simulink model "simulink_part"  (R2016a)
settings: Solver=VariableStepAuto  StartTime=0.0  StopTime=1  RelTol=1e-3
libraries: powerlib x6, powerlib_meascontrol x6
settings Model: Creator=ziad abdelhamed  LastModifiedBy=ziad abdelhamed

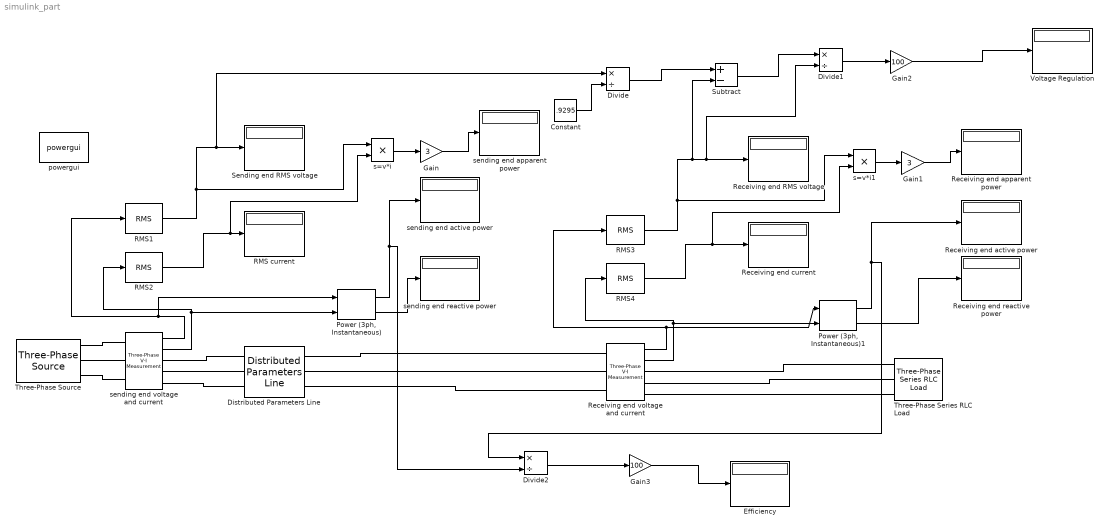
== system simulink_part ==
  Constant : Constant  Value=.9295
  Distributed Parameters Line : powerlib/Elements/Distributed Parameters Line  Phases=3  Frequency=60  Resistance=[.05 .05]  Inductance=[0.97e-3 .99e-3]  Capacitance=[11.5e-9 11.5e-9]  Length=300  x1=[8.73114913702011e-11 617530 617530;376.991118430775 376.991118430775 376.991118430775;1.18918707880175 0.426861843081656 -1.14393448371324]  x2=[1.60089247853505e-10 485242.976182768 485242.976182767;376.991118430775 376.991118430775 376.991118430775;-0.612639506584876 0.174011595737851 -1.39678473105705]  x3=[1.48338818762908e-12 1106.67820606831 1106.67820606832;376.991118430775 376.991118430775 376.991118430775;-2.38866595647793 1.209216979252 -0.361579347542891]  x4=[1.45080507751676e-12 3320.58863195203 3320.58863195202;376.991118430775 376.991118430775 376.991118430775;0.308585693257765 -0.174792776282672 -1.74558910307757]  x5=0.00101224996912818  V1=[8.731e-11 6.175e+05 6.175e+05;377 377 377;1.189 0.4269 -1.144]  V2=[1.601e-10 4.852e+05 4.852e+05;377 377 377;-0.6126 0.174 -1.397]  I1=[1.483e-12 1107 1107;377 377 377;-2.389 1.209 -0.3616]  I2=[1.451e-12 3321 3321;377 377 377;0.3086 -0.1748 -1.746]  nHarmo=1  Measurements=None
  Divide : Product  Inputs=*/
  Divide1 : Product  Inputs=*/
  Divide2 : Product  Inputs=*/
  "Efficiency " : Display
  Gain : Gain  Gain=3
  Gain1 : Gain  Gain=3
  Gain2 : Gain  Gain=100
  Gain3 : Gain  Gain=100
  "Power (3ph, Instantaneous)" : powerlib_meascontrol/Measurements/Power (3ph, Instantaneous)
  "Power (3ph, Instantaneous)1" : powerlib_meascontrol/Measurements/Power (3ph, Instantaneous)
  "RMS current " : Display
  RMS{1..4} (4 alike) : powerlib_meascontrol/Measurements/RMS  TrueRMS=on  Freq=60  RMSInit=0  Ts=0
  Receiving end RMS voltage : Display
  Receiving end active power : Display
  "Receiving end apparent power " : Display
  Receiving end current : Display
  "Receiving end reactive power " : Display
  Receiving end voltage and current : powerlib/Measurements/Three-Phase V-I Measurement  VoltageMeasurement=phase-to-ground  SetLabelV=off  LabelV=Vabc  Vpu=off  VpuLL=off  CurrentMeasurement=yes  SetLabelI=off  LabelI=Iabc  Ipu=off  Pbase=100e6  Vbase=500e3  OutputType=Complex  PhasorSimulation=off  PSBequivalent=0
  Sending end RMS voltage : Display
  Subtract : Sum  Inputs=+-
  Three-Phase Series RLC Load : powerlib/Elements/Three-Phase Series RLC Load  LConnTagsString=A|B|C  Configuration=Y (grounded)  NominalVoltage=500e3  Vabc=[1e3 1e3 1e3]  Vabcp=[1e3 1e3 1e3]  NominalFrequency=60  UnbalancedPower=off  ActivePower=800e6  InductivePower=600e6  CapacitivePower=0  Pabc=[10e3 9e3 11e3]  QLabc=[100 90 110]  QCabc=[100 90 110]  Pabcp=[10e3 9e3 11e3]  QLabcp=[100 90 110]  QCabcp=[100 90 110]  Measurements=None  LoadType=constant Z
  Three-Phase Source : powerlib/Electrical Sources/Three-Phase Source  InternalConnection=Yg  VoltagePhases=off  Voltage=617.53e3  PhaseAngle=16.1  Voltage_phases=[25e3 25e3 25e3]/sqrt(3)  PhaseAngles_phases=[0 -120 +120]  Frequency=60  NonIdealSource=off  SpecifyImpedance=off  Resistance=0.8929  Inductance=16.58e-3  ShortCircuitLevel=100e6  BaseVoltage=25e3  XRratio=7  BusType=swing  Pref=10e3  Qref=0  Prefabc=[10e3, 10e3, 10e3]  Qrefabc=[0, 0, 0]  Qmin=-inf  Qmax=inf
  "Voltage Regulation " : Display
  powergui : powerlib/powergui  Priority=1  SimulationMode=Continuous  SolverType=Tustin/Backward Euler (TBE)  SampleTime=50e-6  frequency=60  SPID=off  DisableSnubberDevices=off  DisableRonSwitches=off  DisableVfSwitches=off  SwTol=0  DisplayEquations=off  Interpol=off  ExternalGateDelay=off  methode=off  Ts=10  FunctionMessages=off  echomessages=off  HookPort=off  EnableUseOfTLC=off  x0status=blocks  frequencyindice=60  Pbase=100e6  ErrMax=1e-4  Iterations=50  UnitsV=kV  UnitsW=MW  buscounter=0  RestoreLinks=warning  ResistiveCurrentMeasurement=off  Frange=[0:2:500]  Ylog=off  Xlog=on  ShowGrid=off  save=off  variable=ZData  structure=0  ZoomFFT=off  StartTime=0.0  cycles=1  DisplayStyle=1  fundamental=60  FreqAxis=off  MaxFrequency=1000  frequencyindicesteady=1  RmsSteady=1  display=off
  s=v*i : Product
  s=v*i1 : Product
  sending end active power : Display
  "sending end apparent power " : Display
  sending end reactive power : Display
  "sending end voltage and current " : powerlib/Measurements/Three-Phase V-I Measurement  VoltageMeasurement=phase-to-ground  SetLabelV=off  LabelV=Vabc  Vpu=off  VpuLL=off  CurrentMeasurement=yes  SetLabelI=off  LabelI=Iabc  Ipu=off  Pbase=100e6  Vbase=500e3  OutputType=Complex  PhasorSimulation=off  PSBequivalent=0
  wires:
  "sending end voltage and current "/1 -> "Power (3ph, Instantaneous)"/1, RMS1/1
  RMS1/1 -> s=v*i/1, Divide/1, Sending end RMS voltage/1
  "sending end voltage and current "/2 -> "Power (3ph, Instantaneous)"/2, RMS2/1
  "Power (3ph, Instantaneous)"/1 -> Divide2/2, sending end active power/1
  "Power (3ph, Instantaneous)"/2 -> sending end reactive power/1
  RMS2/1 -> s=v*i/2, "RMS current "/1
  s=v*i/1 -> Gain/1
  Gain/1 -> "sending end apparent power "/1
  Receiving end voltage and current/1 -> RMS3/1, "Power (3ph, Instantaneous)1"/1
  RMS3/1 -> s=v*i1/1, Subtract/2, Divide1/2, Receiving end RMS voltage/1
  Receiving end voltage and current/2 -> "Power (3ph, Instantaneous)1"/2, RMS4/1
  "Power (3ph, Instantaneous)1"/1 -> Divide2/1, Receiving end active power/1
  "Power (3ph, Instantaneous)1"/2 -> "Receiving end reactive power "/1
  RMS4/1 -> s=v*i1/2, Receiving end current/1
  s=v*i1/1 -> Gain1/1
  Gain1/1 -> "Receiving end apparent power "/1
  Constant/1 -> Divide/2
  Divide/1 -> Subtract/1
  Subtract/1 -> Divide1/1
  Divide1/1 -> Gain2/1
  Gain2/1 -> "Voltage Regulation "/1
  Divide2/1 -> Gain3/1
  Gain3/1 -> "Efficiency "/1
  connections:
  Three-Phase Source/RConn1 -- "sending end voltage and current "/LConn1
  Three-Phase Source/RConn2 -- "sending end voltage and current "/LConn2
  Three-Phase Source/RConn3 -- "sending end voltage and current "/LConn3
  "sending end voltage and current "/RConn3 -- Distributed Parameters Line/LConn3
  "sending end voltage and current "/RConn2 -- Distributed Parameters Line/LConn2
  "sending end voltage and current "/RConn1 -- Distributed Parameters Line/LConn1
  Distributed Parameters Line/RConn3 -- Receiving end voltage and current/LConn3
  Distributed Parameters Line/RConn2 -- Receiving end voltage and current/LConn2
  Distributed Parameters Line/RConn1 -- Receiving end voltage and current/LConn1
  Receiving end voltage and current/RConn1 -- Three-Phase Series RLC Load/LConn1
  Receiving end voltage and current/RConn2 -- Three-Phase Series RLC Load/LConn2
  Receiving end voltage and current/RConn3 -- Three-Phase Series RLC Load/LConn3
